simulink model "dspafxf"  (Simulink 6.0)
settings: Solver=FixedStepDiscrete  StartTime=0.0  StopTime=3.928  RelTol=1e-3
PreLoadFcn:
  | load dspafxf;
values from neighbouring files (symbols this model uses):
  D = var(Noisef)    [lmsxy.m]
undefined symbols (not defined in the file or in its folder): fs_afxf
libraries: dspsrcs4 x3, dspsigops x1
settings Model: CovMetricSettings=d  Creator=don  LastModifiedBy=mkhan  ExtModeTrigMode=oneshot  ExtModeArmWhenConnect=off  SaveTime=off  SaveOutput=off  LimitDataPoints=off  SignalLoggingName=logsOut  IntegerOverflowMsg=none  BlockReductionOpt=off  ZeroCrossControl=DisableAll  ProdHWDeviceType=Microprocessor  TargetHWChar=2  TargetHWWordLengths=8,16,32,32  RTWMathFcnLibMatFile=iso_c_tmw.mat  RTWOptions="-aEnforceIntegerDowncast=1 -aFoldNonRolledExpr=1 -aInlineInvariantSignals=1 -aInlineParameters=0 -aLocalBlockOutputs=1 -aRollThreshold=2 -aGenerateReport=0 -aGenCodeOnly=0 -aRTWVerbose=1 -aForceParamTrailComments=0 -aGenerateComments=1 -aIgnoreCustomStorageClasses=1 -aIncHierarchyInIds=0 -aMaxRTWIdLen=31 -aShowEliminatedStatements=0 -aPrefixModelToSubsysFcnNames=1 -aIncDataTypeInIds=0 -aInlinedPrmAccess=\"Literals\" -aTargetFcnLib=\"iso_c_tmw.mat\" -aGenerateFullHeader=1 -aIsPILTarget=0 -aExtMode=0 -aExtModeStaticAlloc=0 -aExtModeTesting=0 -aExtModeStaticAllocSize=1000000 -aExtModeTransport=0 -aLogVarNameModifier=\"rt_\" -aRTWCAPISignals=0 -aRTWCAPIParams=0"
settings SolverCC: ZeroCrossControl=DisableAll
settings DataIOCC: LimitDataPoints=off  SaveOutput=off  SaveTime=off  SignalLoggingName=logsOut
settings OptimizationCC: BlockReduction=off  BooleanDataType=off  MultiInstanced=off  RollThreshold=2
settings FormatCC: IgnoreBidirectionalLines=off
settings DebuggingCC: IntegerOverflowMsg=none
settings HardwareCC: ProdHWDeviceType=Microprocessor  ShiftRightIntArith=on  TargetHWCharacteristics=InheritFromRTWHook
settings CodeAppCC: FileBanners=off
settings GRTTargetCC: TargetFcnLib=iso_c_tmw.mat  IsERTTarget=off

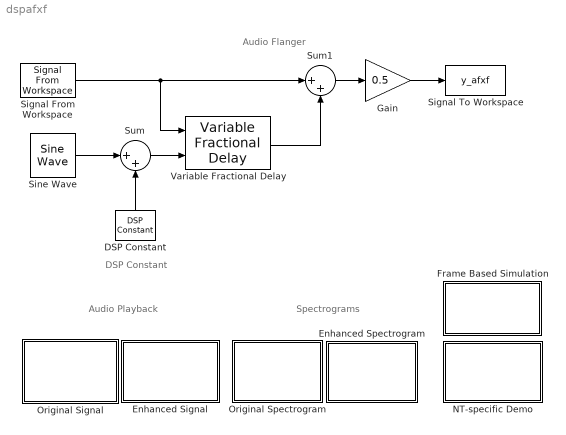
== system dspafxf ==
  note: Audio Playback
  note: Spectrograms
  note: Audio Flanger
  note: DSP Constant
  DSP Constant : dspsrcs4/DSP Constant  Orientation=up  Value=20  SampleMode=Discrete  discreteOutput=Sample-based (interpret vectors as 1-D)  continuousOutput=Sample-based  sampTime=128/fs_afxf  framePeriod=128/fs_afxf  dataType=Inherit from 'Constant value'  wordLen=16  udDataType=sfix(16)  fracBitsMode=Best precision  numFracBits=15  InterpretAs1D=on  Ts=128/fs_afxf  FramebasedOutput=off
  Enhanced Signal : Subsystem
      settings: OpenFcn=if exist('y_afxf','var') & exist('fs_afxf','var'), sound(squeeze(y_afxf),fs_afxf); else errordlg('You must run the simulation first.','Signal Processing Blockset Demo Error'); end
      mask Display: disp('Enhanced\nSignal')
  Enhanced Spectrogram : Subsystem
      settings: OpenFcn=if exist('y_afxf','var') & exist('fs_afxf','var'), figure;specgram(y_afxf,[],fs_afxf);colormap(bone);colorbar; else errordlg('You must run the simulation first.','Signal Processing Blockset Demo Error'); end
      mask Display: disp('Enhanced\nSignal')
  Frame Based Simulation : Subsystem
      mask Type: Frame-Based Simulation Info
      mask Display: disp('Info')
  Gain : Gain  Gain=0.5  SaturateOnIntegerOverflow=on
  NT-specific Demo : Subsystem
      settings: OpenFcn=dspafxf_win32
      mask Type: NT-only Demo
      mask Display: disp('PC/Windows\nDemo')
  Original Signal : Subsystem
      settings: OpenFcn=if exist('x_afxf','var') & exist('fs_afxf','var'), sound(x_afxf,fs_afxf); else errordlg('Data not found in workspace - reload demo model.','Signal Processing Blockset Demo Error'); end
      mask Type: Original Signal
      mask Display: disp('Original\nSignal')
  Original Spectrogram : Subsystem
      settings: OpenFcn=if exist('x_afxf','var') & exist('fs_afxf','var'), figure;specgram(x_afxf,[],fs_afxf);colormap(bone);colorbar; else errordlg('Data not found in workspace - reload demo model.','Signal Processing Blockset Demo Error'); end
      mask Display: disp('Original\nSignal')
  Signal To Workspace : ToWorkspace  VariableName=y_afxf  SampleTime=-1  SaveFormat=Array
  Signal From Workspace : dspsrcs4/Signal From Workspace  X=x_afxf  Ts=1/fs_afxf  nsamps=128  OutputAfterFinalValue=Setting to zero
  Sine Wave : dspsrcs4/Sine Wave  Amplitude=15  Frequency=1/3.934  Phase=pi/4  SampleMode=Discrete  OutComplex=Real  CompMethod=Trigonometric fcn  TableSize=Speed  SampleTime=1/fs_afxf  SamplesPerFrame=128  dataType=double  wordLen=16  udDataType=sfix(16)  fracBitsMode=Best precision  numFracBits=15  ResetState=Restart at time zero
  Sum : Sum  Inputs=|++  SaturateOnIntegerOverflow=on  InputSameDT=on
  Sum1 : Sum  Inputs=|++  SaturateOnIntegerOverflow=on  InputSameDT=on
  Variable Fractional Delay : dspsigops/Variable Fractional Delay  mode=FIR Interpolation  dmax=100  L=8  R=10  alpha=0.5  ic=0
  wires:
  Sum1/1 -> Gain/1
  Variable Fractional Delay/1 -> Sum1/2
  Signal From Workspace/1 -> Sum1/1, Variable Fractional Delay/1
  Sum/1 -> Variable Fractional Delay/2
  Gain/1 -> Signal To Workspace/1
  Sine Wave/1 -> Sum/1
  DSP Constant/1 -> Sum/2

== system dspafxf/Enhanced Signal ==

== system dspafxf/Enhanced Spectrogram ==

== system dspafxf/Frame Based Simulation ==
  note: This simulation of audio flanging employs frame-based processing.
      |
      | By default, the simulation uses 128 samples per frame.
      |
      | If you would like to compare the simulation speed with non-frame
      | based processing, set the "Samples per frame" option to 1 in both
      | the "Signal From Workspace" and "Sine Wave" blocks and set
      | "Sample time" option to 1/fs_afxf in "DSP Constant" block.

== system dspafxf/NT-specific Demo ==

== system dspafxf/Original Signal ==

== system dspafxf/Original Spectrogram ==
